simulink model "myexp7_3"  (R2022a)
settings: Solver=VariableStepAuto  StartTime=0.0  StopTime=10  RelTol=1e-3
libraries: commfilt2 x2, commchan3 x1, commrandsrc3 x1, commsink2 x1, dspfdesign x1, dspstat3 x1, dspsigops x1
settings Model: Creator=惠普  LastModifiedBy=惠普

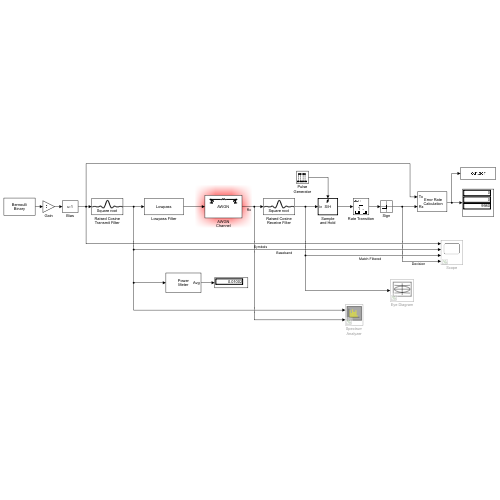
[thumbnail: Simulink's stored preview of the top-level diagram]
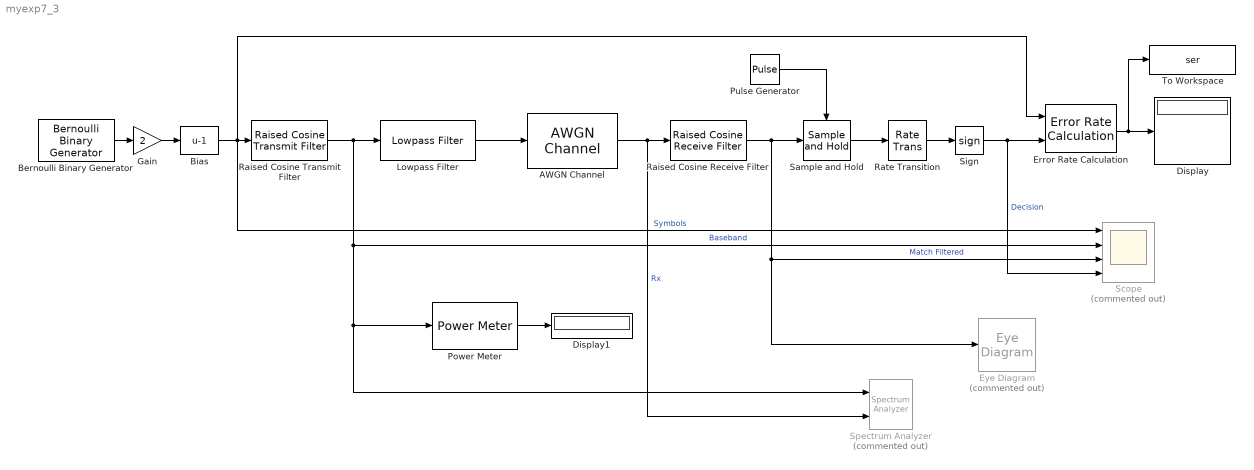
== system myexp7_3 ==
  AWGN Channel : commchan3/AWGN Channel  InputProcessing=Columns as channels (frame based)  seed=137  noiseMode="Signal to noise ratio  (Es/No)"  EbNodB=10  EsNodB=SNR  SNRdB=10  bitsPerSym=1  Ps=0.01  Tsym=1e-3  variance=1
  Bernoulli Binary Generator : commrandsrc3/Bernoulli Binary Generator  ProbabilityOfZero=0.5  SeedSource=Auto  Seed=0  SampleTime=1e-3  SamplesPerFrame=1  OutputDataType=double  SimulateUsing=Interpreted execution
  Bias : Bias  Bias=-1  SaturateOnIntegerOverflow=off
  Display : Display
  Display1 : Display
  Error Rate Calculation : commsink2/Error Rate Calculation  N=21  st_delay=0  cp_mode=Entire frame  subframe=[]  PMode=Port  WsName=ErrorVec  RsMode2=off  stop=off  numErr=100  maxBits=1e6
  Eye Diagram : EyeDiagram  Commented=on
  Gain : Gain  Gain=2
  Lowpass Filter : dspfdesign/Lowpass Filter  FilterType=FIR  DesignForMinimumOrder=on  FilterOrder=50  PassbandFrequency=0.7e3  StopbandFrequency=0.8e3  PassbandRipple=0.1  StopbandAttenuation=40  InheritSampleRate=off  SampleRate=100e3  SimulateUsing=Interpreted execution  roundingMode=Floor  coeffsDataTypeStr=fixdt(1,16)
  Power Meter : dspstat3/Power Meter  Measurement=Average power  WindowLength=10e3  ReferenceLoad=1  OutputPowerUnits=Watts  SimulateUsing=Code generation
      settings: SourceProductBaseCode=DS
  Pulse Generator : DiscretePulseGenerator  Period=100  PhaseDelay=59  SampleTime=10e-6
  Raised Cosine Receive Filter : commfilt2/Raised Cosine Receive Filter  filtType=Square root  R=0.5  filtSpan=10  N=100  downFactor=1  downOffset=0  filterGain=1  InputProcessing=Columns as channels (frame based)  RateOptions=Allow multirate processing  framing=Mute  checkCoeff=off  variableName=rcRxFilt  currentFiltSpan=10  D=5  inputOffset=0  sampMode=Mute  saveAsFlag=0  rateMode=Downsampling  checkGain=Normalized  launchFVT=on  roundingMode=Floor  overflowMode=off  coeffDataTypeStr=Inherit: Same word length as input  coeffMin=[]  coeffMax=[]  coeffLastDataTypeStr=Inherit: Same word length as input  accumDataTypeStr=Inherit: Same as product output  accumLastDataTypeStr=Inherit: Same as product output  outputDataTypeStr=Inherit: Same as accumulator  outputMin=[]  outputMax=[]  outputLastDataTypeStr=Inherit: Same as accumulator
  Raised Cosine Transmit Filter : commfilt2/Raised Cosine Transmit Filter  filtType=Square root  R=0.5  filtSpan=10  N=100  filterGain=1  InputProcessing=Columns as channels (frame based)  RateOptions=Allow multirate processing  framing=Mute  checkCoeff=off  variableName=rcTxFilt  checkGain=Normalized  sampMode=Mute  saveAsFlag=0  currentFiltSpan=10  D=(10)/2  launchFVT=on  roundingMode=Floor  overflowMode=off  coeffDataTypeStr=Inherit: Same word length as input  coeffMin=[]  coeffMax=[]  coeffLastDataTypeStr=Inherit: Same word length as input  outputDataTypeStr=Inherit: Same as accumulator  outputMin=[]  outputMax=[]  outputLastDataTypeStr=Inherit: Same as accumulator
  Rate Transition : RateTransition  OutPortSampleTime=1e-3
  Sample and Hold : dspsigops/Sample and Hold  trig=Rising edge  initCond=0  latchinput=off
  Scope : Scope  Commented=on  NumInputPorts=4
  Sign : Signum
  Spectrum Analyzer : SpectrumAnalyzer  Commented=on  NumInputPorts=2
  To Workspace : ToWorkspace  VariableName=ser  SampleTime=-1
      settings: MaxDataPoints=1
  wires:
  Bernoulli Binary Generator/1 -> Gain/1
  Gain/1 -> Bias/1
  Bias/1 -> Error Rate Calculation/1, Scope/1, Raised Cosine Transmit Filter/1  "Symbols"
  AWGN Channel/1 -> Spectrum Analyzer/2, Raised Cosine Receive Filter/1  "Rx"
  Raised Cosine Receive Filter/1 -> Eye Diagram/1, Scope/3, Sample and Hold/1  "Match Filtered"
  Pulse Generator/1 -> Sample and Hold/Trigger
  Sample and Hold/1 -> Rate Transition/1
  Rate Transition/1 -> Sign/1
  Sign/1 -> Scope/4, Error Rate Calculation/2  "Decision"
  Error Rate Calculation/1 -> To Workspace/1, Display/1
  Raised Cosine Transmit Filter/1 -> Scope/2, Spectrum Analyzer/1, Power Meter/1, Lowpass Filter/1  "Baseband"
  Lowpass Filter/1 -> AWGN Channel/1
  Power Meter/1 -> Display1/1
